simulink model "Practica5_T_Simulink"  (R2022b)
settings: Solver=VariableStepAuto  StartTime=0.0  StopTime=0.01  MaxStep=0.00001  RelTol=1e-3
values from neighbouring files (symbols this model uses):
  C = 10e-6    (= 1e-05)    [Parametros_Practica5.m]    (also in Practica5.m)
  d = 0.4    [Parametros_Practica5.m]    (also in Practica5.m)
  L = 2e-3    (= 0.002)    [Parametros_Practica5.m]    (also in Practica5.m)
  R = 10    [Parametros_Practica5.m]    (also in Practica5.m)
  Uin = 32    [Parametros_Practica5.m]    (also in Practica5.m)
settings Model: Creator=52466  LastModifiedBy=52466

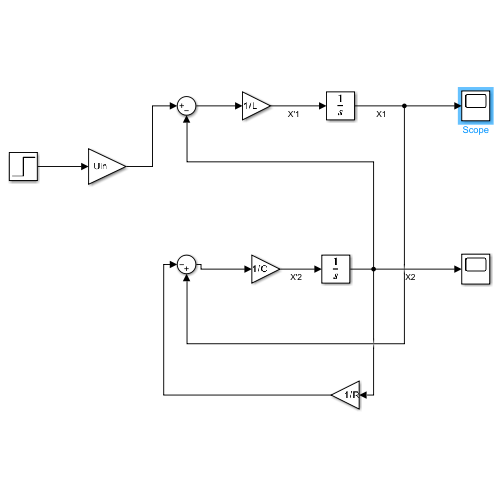
[thumbnail: Simulink's stored preview of the top-level diagram]
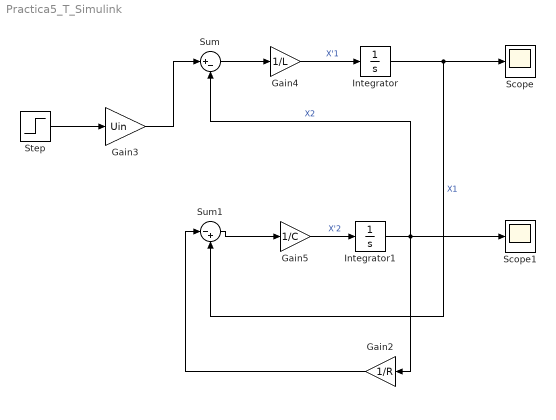
== system Practica5_T_Simulink ==
  Gain2 : Gain  Gain=1/R
  Gain3 : Gain  Gain=Uin
  Gain4 : Gain  Gain=1/L
  Gain5 : Gain  Gain=1/C
  Integrator : Integrator
  Integrator1 : Integrator
  Scope : Scope
  Scope1 : Scope
  Step : Step  Time=0  After=d  SampleTime=0
  Sum : Sum  Inputs=|+-
  Sum1 : Sum  Inputs=|-+
  wires:
  Integrator/1 -> Sum1/2, Scope/1  "X1"
  Sum1/1 -> Gain5/1
  Integrator1/1 -> Sum/2, Scope1/1, Gain2/1  "X2"
  Gain2/1 -> Sum1/1
  Gain3/1 -> Sum/1
  Sum/1 -> Gain4/1
  Gain4/1 -> Integrator/1  "X'1"
  Gain5/1 -> Integrator1/1  "X'2"
  Step/1 -> Gain3/1
